simulink model "slm6"  (R2018a)
settings: Solver=VariableStepAuto  StartTime=0.0  StopTime=10.0  RelTol=1e-9
values from neighbouring files (symbols this model uses):
  b1 = 2.817    [setup.m]
  b2 = 1227.0    (= 1227)    [setup.m]
  b3 = 0.2090    (= 0.209)    [setup.m]
  b4 = 4.560    (= 4.56)    [setup.m]
  b5 = 1.678    [setup.m]
  b6 = -0.4571    [setup.m]
  c1 = 116    [setup.m]
  c2 = .349    (= 0.349)    [setup.m]
  k1 = 3930    [setup.m]
  k2 = 5720    [setup.m]
  k3 = 123    [setup.m]
  m = 1.2    [setup.m]
  W = 88    [setup.m]
settings Model: Creator=Pranav Maddula  LastModifiedBy=Pranav Maddula

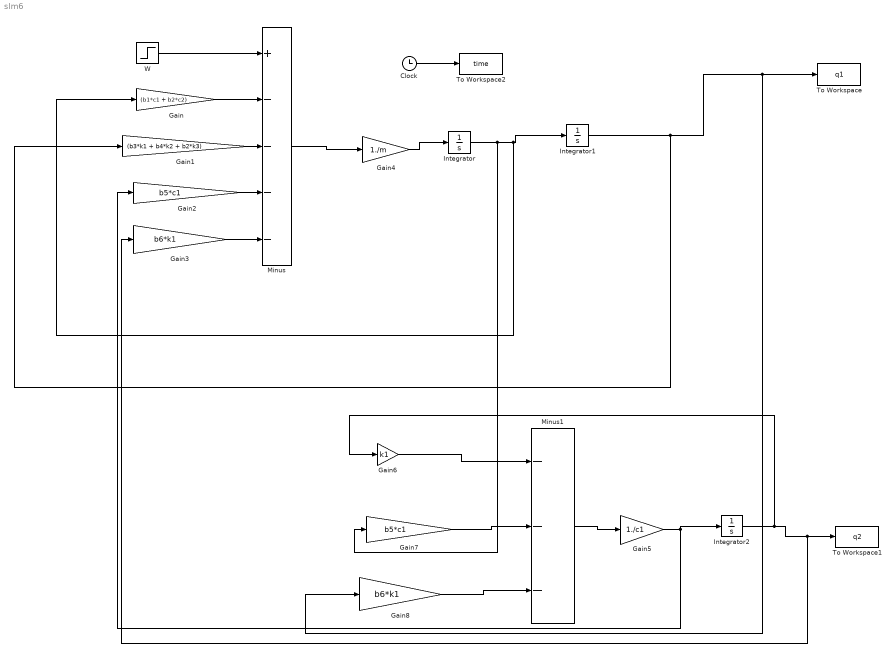
== system slm6 ==
  Clock : Clock
  Gain : Gain  Gain=(b1*c1 + b2*c2)
  Gain1 : Gain  Gain=(b3*k1 + b4*k2 + b2*k3)
  Gain2 : Gain  Gain=b5*c1
  Gain3 : Gain  Gain=b6*k1
  Gain4 : Gain  Gain=1./m
  Gain5 : Gain  Gain=1./c1
  Gain6 : Gain  Gain=k1
  Gain7 : Gain  Gain=b5*c1
  Gain8 : Gain  Gain=b6*k1
  Integrator : Integrator
  Integrator1 : Integrator  InitialCondition=.069
  Integrator2 : Integrator
  Minus : Sum  Inputs=+----
  Minus1 : Sum  Inputs=---
  To Workspace : ToWorkspace  VariableName=q1  SampleTime=-1
  To Workspace1 : ToWorkspace  VariableName=q2  SampleTime=-1
  To Workspace2 : ToWorkspace  VariableName=time  SampleTime=-1
  "W " : Step  After=W  SampleTime=0
  wires:
  "W "/1 -> Minus/1
  Integrator/1 -> Gain7/1, Gain/1, Integrator1/1
  Minus/1 -> Gain4/1
  Gain4/1 -> Integrator/1
  Integrator1/1 -> Gain1/1, Gain8/1, To Workspace/1
  Integrator2/1 -> Gain6/1, Gain3/1, To Workspace1/1
  Gain5/1 -> Integrator2/1, Gain2/1
  Minus1/1 -> Gain5/1
  Gain8/1 -> Minus1/3
  Gain7/1 -> Minus1/2
  Gain6/1 -> Minus1/1
  Gain/1 -> Minus/2
  Gain1/1 -> Minus/3
  Gain2/1 -> Minus/4
  Gain3/1 -> Minus/5
  Clock/1 -> To Workspace2/1
